simulink library "HEMERO"  (Simulink 3.00)
values from neighbouring files (symbols this model uses):
  K1 = 0.5    [ejh64.m]    (also in ejh65.m)
  K2 = 0.8    [ejh64.m]    (also in ejh65.m)
  x_camino = 0:0.01:10    [ejh64.m]    (also in ejh65.m)
  y_camino = x_camino.^2    [ejh64.m]    (also in ejh65.m)
undefined symbols (not defined in the file or in its folder): magnitude, nonlinear
libraries: simulink_extras x12, HEMERO x9, simulink3 x6, dspstat x4
(part 1 of 9)
settings Model: LastModifiedBy=Administrador

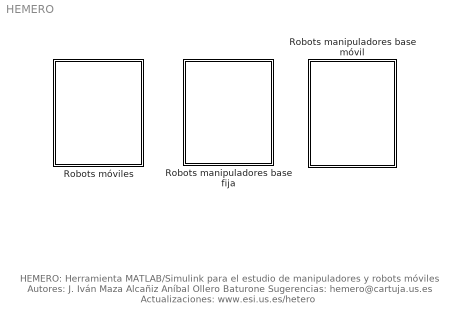
== system HEMERO ==
  note: HEMERO: Herramienta MATLAB/Simulink para el estudio de
      | manipuladores y robots móviles
      | Autores:
      | J. Iván Maza Alcañiz
      | Aníbal Ollero Baturone
      |
      | Sugerencias: hemero@cartuja.us.es
      | Actualizaciones: www.esi.us.es/hetero
  Robots manipuladores base fija : Subsystem
  Robots manipuladores base móvil : Subsystem
  Robots móviles : Subsystem

== system HEMERO/Robots manipuladores base fija ==
  Control basado en el modelo : Subsystem
  Modelo Dinámico : Subsystem

== system HEMERO/Robots manipuladores base móvil ==
  Modelo Dinámico : Subsystem

== system HEMERO/Robots móviles ==
  Control de robots móviles : Subsystem
  Modelos cinemáticos directos : Subsystem
  Modelos cinemáticos inversos : Subsystem

== system HEMERO/Robots manipuladores base fija/Control basado en el modelo ==
  Control Adaptativo : Subsystem
  Control con aprendizaje : Subsystem
  Par Computado : Subsystem

== system HEMERO/Robots manipuladores base fija/Modelo Dinámico ==
  Ejemplos : Subsystem
  Inversa de la matriz de masas : Subsystem  mask(Inversa de la matriz de masas){dyn=}
      mask prompts: dyn "Matriz de parámetros cinemáticos y dinámicos:"
      mask help: Este bloque calcula el producto de la inversa de la matriz de masas por el vector columna In que se le pasa como entrada.
  Modelo de fricciones : Subsystem  mask(Modelo de fricciones (viscosa y de Coriolis)){G=, b=, tcp=, tcm=}
      mask prompts: G "Factores de reducción (G):"; b "Fricciones viscosas, referidas al motor:"; tcp "Fricciones de Coulomb (rotación +), referidas al motor:"; tcm "Fricciones de Coulomb (rotación -), referidas al motor:"
      mask help:
      | Este bloque calcula el par correspondiente a la fricciones viscosa y de Coulomb. Para ello se emplea un determinado modelo para dichas fricciones:
      |            B·q' + Tc + ,  si q'>0
      |            B·q' + Tc - ,  si q'<0
      mask Display:
      | disp('B·q'' + Tc + ,  si q''>0\n')
      | disp('\nB·q'' + Tc - ,  si q''<0')
  Par total : Subsystem  mask(Par total){dyn=, grav=}
      mask prompts: dyn "Matriz de parámetros cinemáticos y dinámicos:"; grav "Vector aceleración de la gravedad:"
      mask help: Este bloque calcula el par total. Se incluye un modelo de las fricciones igual al empleado en el bloque "Modelo de fricciones". Si se quiere eliminar este término de fricciones para usar un modelo distinto, basta con hacer nulas las columnas 18, 19 y 20 de la matriz de parámetros cinemáticos y dinámicos.
  Trayectorias articulares : Subsystem  mask(Trayectorias articulares){dyn=, grav=, inivel=, inipos=}
      mask prompts: dyn "Matriz de parámetros cinemáticos y dinámicos:"; grav "Vector aceleración de la gravedad:"; inivel "Velocidades articulares iniciales:"; inipos "Posiciones articulares iniciales:"
      mask help: Se calculan las trayectorias articulares (posiciones, velocidades y aceleraciones articulares) a partir de los pares aplicados al manipulador.
  Término Vm de Coriolis : Subsystem  mask(Producto por el término Vm){dyn=}
      mask prompts: dyn "Matriz de parámetros cinemáticos y dinámicos:"
      mask help: Este bloque calcula el producto del término Vm por el vector columna In que se le pasa como entrada.
  Término de la matriz de masas : Subsystem  mask(Término asociado a la matriz de masas){dyn=}
      mask prompts: dyn "Matriz de parámetros cinemáticos y dinámicos:"
      mask help: Este bloque calcula el par correspondiente al término en el que aparece la matriz de masas.
  Términos gravitatorios : Subsystem  mask(Término gravitatorio){dyn=, grav=}
      mask prompts: dyn "Matriz de parámetros cinemáticos y dinámicos:"; grav "Vector aceleración de la gravedad:"
      mask help: Este bloque calcula el par correspondiente al término gravitatorio.
  Términos centrífugos y de Coriolis : Subsystem  mask(Términos centrífugos y de Coriolis){dyn=}
      mask prompts: dyn "Matriz de parámetros cinemáticos y dinámicos:"
      mask help: Este bloque calcula el par correspondiente a los términos centrífugos y de Coriolis.

== system HEMERO/Robots manipuladores base móvil/Modelo Dinámico ==
  Ejemplos : Subsystem
  Inversa de la matriz de masas : Subsystem  mask(Inversa de la matriz de masas){dyn=}
      mask prompts: dyn "Matriz de parámetros cinemáticos y dinámicos:"
      mask help: Este bloque calcula el producto de la inversa de la matriz de masas por el vector columna In que se le pasa como entrada, para el caso de base móvil.
  Modelo de fricciones : Subsystem  mask(Modelo de fricciones (viscosa y de Coriolis)){G=, b=, tcp=, tcm=}
      mask prompts: G "Factores de reducción (G):"; b "Fricciones viscosas, referidas al motor:"; tcp "Fricciones de Coulomb (rotación +), referidas al motor:"; tcm "Fricciones de Coulomb (rotación -), referidas al motor:"
      mask help:
      | Este bloque calcula el par correspondiente a la fricciones viscosa y de Coulomb. Para ello se emplea un determinado modelo para dichas fricciones:
      |            B·q' + Tc + ,  si q'>0
      |            B·q' + Tc - ,  si q'<0
      mask Display:
      | disp('B·q'' + Tc + ,  si q''>0\n')
      | disp('\nB·q'' + Tc - ,  si q''<0')
  Par total : Subsystem  mask(Par total){dyn=, grav=}
      mask prompts: dyn "Matriz de parámetros cinemáticos y dinámicos:"; grav "Vector aceleración de la gravedad:"
      mask help: Este bloque calcula el par total para el caso de base móvil. Se incluye un modelo de las fricciones igual al empleado en el bloque "Modelo de fricciones". Si se quiere eliminar este término de fricciones para usar un modelo distinto, basta con hacer nulas las columnas 18, 19 y 20 de la matriz de parámetros cinemáticos y dinámicos.
  Trayectorias articulares : Subsystem  mask(Trayectorias articulares){dyn=, grav=, inivel=, inipos=}
      mask prompts: dyn "Matriz de parámetros cinemáticos y dinámicos:"; grav "Vector aceleración de la gravedad:"; inivel "Velocidades articulares iniciales:"; inipos "Posiciones articulares iniciales:"
      mask help: Calcula las trayectorias articulares (posiciones, velocidades y aceleraciones articulares) a partir de los pares aplicados al manipulador, para el caso de base móvil.
  Término Vm de Coriolis : Subsystem  mask(Producto por el término Vm){dyn=}
      mask prompts: dyn "Matriz de parámetros cinemáticos y dinámicos:"
      mask help: Este bloque calcula el producto del término Vm por el vector columna In que se le pasa como entrada, para el caso de base móvil.
  Término de la matriz de masas : Subsystem  mask(Término asociado a la matriz de masas){dyn=}
      mask prompts: dyn "Matriz de parámetros cinemáticos y dinámicos:"
      mask help: Este bloque calcula el par correspondiente al término en el que aparece la matriz de masas para el caso de base móvil.
  Términos gravitatorios : Subsystem  mask(Término gravitatorio){dyn=, grav=}
      mask prompts: dyn "Matriz de parámetros cinemáticos y dinámicos:"; grav "Vector aceleración de la gravedad:"
      mask help: Este bloque calcula el par correspondiente al término gravitatorio para el caso de base móvil.
  Términos centrífugos y de Coriolis : Subsystem  mask(Términos centrífugos y de Coriolis){dyn=}
      mask prompts: dyn "Matriz de parámetros cinemáticos y dinámicos:"
      mask help: Este bloque calcula el par correspondiente a los términos centrífugos y de Coriolis para el caso de base móvil.

== system HEMERO/Robots móviles/Control de robots móviles ==
  Métodos geométricos : Subsystem
  Métodos basados en Teoría de Control : Subsystem

== system HEMERO/Robots móviles/Modelos cinemáticos directos ==
  Modelo directo Bicicleta : Subsystem  mask(Modelo directo bicicleta){x_ini=, y_ini=, phi_ini=, alpha_ini=, c=, l=}
      mask prompts: x_ini "Coordenada x inicial del móvil:"; y_ini "Coordenada y inicial del móvil:"; phi_ini "Valor inicial de la orientación del vehículo (rad):"; alpha_ini "Valor inicial de la orientación de la rueda delantera (rad):"; c "Radio de las ruedas"; l "Longitud entre rueda delantera y trasera:"
      mask help: Calcula las coordenadas y orientación del vehículo a partir de las variables de control wt (velocidad angular de rotación de la rueda delantera sobre si misma) y walpha (velocidad angular de giro de la rueda delantera).
  Modelo directo Config. Síncrona : Subsystem  mask(Modelo directo config. síncrona){x_ini=, y_ini=, phi_ini=}
      mask prompts: x_ini "Coordenada x inicial del móvil:"; y_ini "Coordenada y inicial del móvil:"; phi_ini "Valor inicial de la orientación del vehículo (rad):"
      mask help: Calcula las coordenadas y orientación del vehículo a partir de las variables de control v y w que son las velocidades lineal y angular respectivamente del vehículo.
  Modelo directo Guiado Diferencial : Subsystem  mask(Modelo directo guiado diferencial){x_ini=, y_ini=, phi_ini=, c=, b=}
      mask prompts: x_ini "Coordenada x inicial del móvil:"; y_ini "Coordenada y inicial del móvil:"; phi_ini "Valor inicial de la orientación del vehículo (rad):"; c "Radio de las ruedas:"; b "Distancia entre las ruedas :"
      mask help: Calcula las coordenadas y orientación del vehículo a partir de las variables de control wi y wd que son las velocidades angulares de las ruedas izquierda y derecha respectivamente.
  Modelo directo Triciclo Clásico : Subsystem  mask(Modelo directo triciclo clásico){x_ini=, y_ini=, phi_ini=, alpha_ini=, c=, l=}
      mask prompts: x_ini "Coordenada x inicial del móvil:"; y_ini "Coordenada y inicial del móvil:"; phi_ini "Valor inicial de la orientación del vehículo (rad):"; alpha_ini "Valor inicial de la orientación de la rueda delantera (rad):"; c "Radio de las ruedas"; l "Longitud entre rueda delantera y traseras:"
      mask help: Calcula las coordenadas y orientación del vehículo a partir de las variables de control wt (velocidad angular de rotación de la rueda delantera sobre si misma) y walpha (velocidad angular de giro de la rueda delantera).

== system HEMERO/Robots móviles/Modelos cinemáticos inversos ==
  Modelo inverso Bicicleta : Subsystem  mask(Modelo inverso de la bicicleta){l=}
      mask prompts: l "Distancia entre la rueda delantera y la rueda trasera:"
      mask help: A partir de las coordenadas (x,y) de la trayectoria de la bicicleta en función del tiempo, este bloque calcula las correspondientes variables de control vt (velocidad lineal de la rueda delantera) y walpha (velocidad angular de giro de la rueda delantera). Asimismo, también calcula el ángulo (alpha) de orientación de la rueda delantera y el ángulo (phi) de orientación del vehículo.
  Modelo inverso Config. Síncrona : Subsystem
      mask Type: Modelo inverso de la configuración síncrona
      mask Description: A partir de las coordenadas (x,y) de la trayectoria del vehículo en función del tiempo, este bloque calcula las correspondientes variables de control v y w que son las velocidades lineal y angular del vehículo. Asimismo, también se calcula la orientación (phi) del vehículo.
  Modelo inverso Guiado Diferencial : Subsystem  mask(Modelo inverso guiado diferencial){b=, c=}
      mask prompts: b "Vía del vehículo:"; c "Radio de las ruedas:"
      mask help: A partir de las coordenadas (x,y) de la trayectoria del vehículo en función del tiempo, este bloque calcula las correspondientes variables de control wi y wd que son las velocidades angulares de giro de las ruedas izquierda y derecha respectivamente.
  Modelo inverso Triciclo Clasico : Subsystem  mask(Modelo inverso del triciclo clasico){l=}
      mask prompts: l "Distancia entre la rueda delantera y las ruedas traseras:"
      mask help: A partir de las coordenadas (x,y) de la trayectoria del triciclo en función del tiempo, este bloque calcula las correspondientes variables de control vt (velocidad lineal de la rueda delantera) y walpha (velocidad angular de giro de la rueda delantera). Asimismo, también calcula el ángulo (alpha) de orientación de la rueda delantera y el ángulo (phi) de orientación del vehículo.

== system HEMERO/Robots manipuladores base fija/Control basado en el modelo/Control Adaptativo ==
  Control de inercia adaptativo : Subsystem  mask(Cálcula los parámetros para el control de inercia adaptativo){dyn=, gamma=, a=, grav=, m_inicial=, b_inicial=, tcp_inicial=, tcm_inicial=}
      mask prompts: dyn "Matriz de parámetros cinemáticos y dinámicos:"; gamma "Matriz gamma:"; a "Matriz A:"; grav "Vector aceleración de la gravedad:"; m_inicial "Estimaciones de las masas:"; b_inicial "Estimaciones de las fricciones viscosas:"; tcp_inicial "Estimaciones de las fricciones de Coulomb (rotación +):"; tcm_inicial "Estimaciones de las fricciones de Coulomb (rotación -):"
      mask help: Este bloque calcula en cada instante las estimaciones de las masas y fricciones de un manipulador según el esquema de control de inercia adaptativo. Asimismo, devuelve el término Y(·)*estim correspondiente a uno de los sumandos que componen el par de control en dicho esquema.
  Ejemplos : Subsystem
  Inversa de la matriz de masas : Subsystem  mask(Inversa de la matriz de masas){dyn=}
      mask prompts: dyn "Matriz de parámetros cinemáticos y dinámicos:"
      mask help: Este bloque calcula el producto de la inversa de la matriz de masas por el vector columna In que se le pasa como entrada. Dispone de una entrada para proporcionarle las estimaciones de las masas en cada instante.
      mask Display:
      | plot([0.05 0.95],[0.05 0.95])
      | plot([0.8 0.95],[0.7 0.95])
      | plot([0.7 0.95],[0.8 0.95])
  Modelo de fricciones : Subsystem  mask(Modelo estimado de fricciones (viscosa y de Coriolis)){G=, b=, tcp=, tcm=}
      mask prompts: G "Factores de reducción (G):"; b "Fricciones viscosas iniciales, referidas al motor:"; tcp "Fricciones de Coulomb (rot +) iniciales, referidas al motor:"; tcm "Fricciones de Coulomb (rot -) iniciales, referidas al motor:"
      mask help:
      | Este bloque calcula el par correspondiente a la fricciones viscosa y de Coulomb. Para ello se emplea un determinado modelo para dichas fricciones:
      |            b·q' + tcp ,  si q'>0
      |            b·q' + tcm ,  si q'<0
      | Dispone de entradas para pasarle las estimaciones de las fricciones en cada instante.
      mask Display:
      | disp('B·q'' + Tc + ,  si q''>0\n')
      | disp('\nB·q'' + Tc - ,  si q''<0')
      | plot([0.05 0.95],[0.05 0.95])
      | plot([0.8 0.95],[0.7 0.95])
      | plot([0.78 0.95],[0.88 0.95])
  Término Vm de Coriolis : Subsystem  mask(Término estimado asociado a la matriz de masas){dyn=}
      mask prompts: dyn "Matriz inicial de parámetros cinemáticos y dinámicos:"
      mask help: Este bloque calcula el par correspondiente al término en el que aparece la matriz de masas. Dispone de una entrada para proporcionarle las estimaciones de las masas en cada instante.
      mask Display:
      | plot([0.05 0.95],[0.05 0.95])
      | plot([0.8 0.95],[0.7 0.95])
      | plot([0.7 0.95],[0.8 0.95])
  Término de la matriz de masas : Subsystem  mask(Término estimado asociado a la matriz de masas){dyn=}
      mask prompts: dyn "Matriz inicial de parámetros cinemáticos y dinámicos:"
      mask help: Este bloque calcula el par correspondiente al término en el que aparece la matriz de masas. Dispone de una entrada para proporcionarle las estimaciones de las masas en cada instante.
      mask Display:
      | plot([0.05 0.95],[0.05 0.95])
      | plot([0.8 0.95],[0.7 0.95])
      | plot([0.7 0.95],[0.8 0.95])
  Términos gravitatorios : Subsystem  mask(Término gravitatorio estimado){dyn=, grav=}
      mask prompts: dyn "Matriz inicial de parámetros cinemáticos y dinámicos:"; grav "Vector aceleración de la gravedad:"
      mask help: Este bloque calcula el par correspondiente al término gravitatorio. Dispone de una entrada para proporcionarle las estimaciones de las masas en cada instante.
      mask Display:
      | plot([0.05 0.95],[0.05 0.95])
      | plot([0.8 0.95],[0.7 0.95])
      | plot([0.7 0.95],[0.8 0.95])
  Términos centrífugos y de Coriolis : Subsystem  mask(Términos centrífugos y de Coriolis estimados){dyn=}
      mask prompts: dyn "Matriz inicial de parámetros cinemáticos y dinámicos:"
      mask help: Este bloque calcula el par correspondiente a los términos centrífugos y de Coriolis. Dispone de una entrada para proporcionarle las estimaciones de las masas en cada instante.
      mask Display:
      | plot([0.05 0.95],[0.05 0.95])
      | plot([0.8 0.95],[0.7 0.95])
      | plot([0.7 0.95],[0.8 0.95])

== system HEMERO/Robots manipuladores base fija/Control basado en el modelo/Control con aprendizaje ==
  Ejemplos : Subsystem
  Par realimentado aprendido : Subsystem  mask(Calcula por aprendizaje el par que hay que añadir a la ley de control){dyn=, Kp=, Kv=, mu=, tfinal=}
      mask prompts: dyn "Matriz de parámetros cinemáticos y dinámicos:"; Kp "Matriz Kp:"; Kv "Matriz Kv:"; mu "Constante mu:"; tfinal "Tiempo final de la simulación:"

== system HEMERO/Robots manipuladores base fija/Control basado en el modelo/Par Computado ==
  Control PD : Subsystem  mask(Controlador PD){Kp=, Kv=}
      mask prompts: Kp "Introduzca la matriz Kp:"; Kv "Introduzca la matriz Kv:"
      mask help: Calcula el par tau_r correspondiente a la técnica del par computado usando un controlador PD.
  Control PID : Subsystem  mask(Controlador PID){Kp=, Kv=, Ki=}
      mask prompts: Kp "Introduzca la matriz Kp:"; Kv "Introduzca la matriz Kv:"; Ki "Introduzca la matriz Ki:"
      mask help: Calcula el par tau_r correspondiente a la técnica del par computado usando un controlador PID.
  Ejemplos : Subsystem

== system HEMERO/Robots manipuladores base fija/Modelo Dinámico/Ejemplos ==
  Ejemplo H.4.2 : Subsystem
  Ejemplo H.4.4a : Subsystem
  Ejemplo H.4.4b : Subsystem
  Ejemplo H.4.4c : Subsystem

== system HEMERO/Robots manipuladores base fija/Modelo Dinámico/Inversa de la matriz de masas ==
  q : Inport  Port=1  PortWidth=-1  SampleTime=-1  DataType=auto
      settings: SignalType=auto
  In : Inport  Port=2  PortWidth=-1  SampleTime=-1  DataType=auto
      settings: SignalType=auto
  Masas : S-Function  FunctionName=sminv  Parameters=dyn  PortCounts=[]  SFunctionModules=''
  Mux : Mux  Inputs=2
      settings: DisplayOption=none
  M(q)^(-1) · In : Outport  Port=1  InitialOutput=0
  wires:
  Masas/1 -> M(q)^(-1) · In/1
  In/1 -> Mux/2
  q/1 -> Mux/1
  Mux/1 -> Masas/1

== system HEMERO/Robots manipuladores base fija/Modelo Dinámico/Modelo de fricciones ==
  q' : Inport  Port=1  PortWidth=-1  SampleTime=-1  DataType=auto
      settings: SignalType=auto
  Fricciones : S-Function  FunctionName=sfriction  Parameters=G,b,tcp,tcm  PortCounts=[]  SFunctionModules=''
  tau_f : Outport  Port=1  InitialOutput=0
  wires:
  Fricciones/1 -> tau_f/1
  q'/1 -> Fricciones/1

== system HEMERO/Robots manipuladores base fija/Modelo Dinámico/Par total ==
  q : Inport  Port=1  PortWidth=-1  SampleTime=-1  DataType=auto
      settings: SignalType=auto
  q' : Inport  Port=2  PortWidth=-1  SampleTime=-1  DataType=auto
      settings: SignalType=auto
  q'' : Inport  Port=3  PortWidth=-1  SampleTime=-1  DataType=auto
      settings: SignalType=auto
  fext : Inport  Port=4  PortWidth=-1  SampleTime=-1  DataType=auto
      settings: SignalType=auto
  Mux : Mux  Inputs=4
      settings: DisplayOption=none
  Par total : S-Function  FunctionName=srne  Parameters=dyn,grav  PortCounts=[]  SFunctionModules=''
  M(q)·q'' + V (q,q') + G(q) + F(q') : Outport  Port=1  InitialOutput=0
  wires:
  Par total/1 -> M(q)·q'' + V (q,q') + G(q) + F(q')/1
  Mux/1 -> Par total/1
  q''/1 -> Mux/3
  q'/1 -> Mux/2
  q/1 -> Mux/1
  fext/1 -> Mux/4

== system HEMERO/Robots manipuladores base fija/Modelo Dinámico/Trayectorias articulares ==
  note: q
  note: q''
  note: q'
  tau : Inport  Port=1  PortWidth=-1  SampleTime=-1  DataType=auto
      settings: SignalType=auto
  Integrator : Integrator  ExternalReset=none  InitialConditionSource=internal  InitialCondition=inivel(:)  LimitOutput=off  UpperSaturationLimit=inf  LowerSaturationLimit=-inf  ShowSaturationPort=off  ShowStatePort=off  AbsoluteTolerance=auto
  Integrator1 : Integrator  ExternalReset=none  InitialConditionSource=internal  InitialCondition=inipos(:)  LimitOutput=off  UpperSaturationLimit=inf  LowerSaturationLimit=-inf  ShowSaturationPort=off  ShowStatePort=off  AbsoluteTolerance=auto
  Inversa de la matriz de masas : Subsystem  mask(Término de Coriolis){dyn=dyn}
      mask prompts: dyn "Matriz de parámetros dinámicos:"
      mask help: Este bloque devuelve el par correspondiente al término de Coriolis.
      mask Help: A este bloque hay que darle tres parámetros: 1) La matriz de parámetros dinámicos del manipulador de acuerdo con el formato que se explica en la sección "dyn" del Apéndice, 2) Un vector columna correspondiente a la aceleración de la gravedad, y 3) Un vector columna correspondiente a las fuerzas externas.
  Modelo de fricciones : Subsystem  mask(Modelo de fricciones (viscosa y de Coriolis)){G=dyn (:,17), b=dyn (:,18), tcp=dyn (:,19), tcm=dyn (:,20)}
      mask prompts: G "Factores de reducción (G):"; b "Fricciones viscosas, referidas al motor:"; tcp "Fricciones de Coulomb (rotación +), referidas al motor:"; tcm "Fricciones de Coulomb (rotación -), referidas al motor:"
      mask help:
      | Este bloque calcula el par correspondiente a la fricciones viscosa y de Coulomb. Para ello se emplea un determinado modelo para dichas fricciones:
      |            B·q' + Tc + ,  si q'>0
      |            B·q' + Tc - ,  si q'<0
      mask Display:
      | disp('B·q'' + Tc + ,  si q''>0\n')
      | disp('\nB·q'' + Tc - ,  si q''<0')
  Sum : Sum  Inputs=+---  SaturateOnIntegerOverflow=on
  Términos gravitatorios : Subsystem  mask(Término de Coriolis){dyn=dyn, grav=grav}
      mask prompts: dyn "Matriz de parámetros dinámicos:"; grav "Vector aceleración de la gravedad:"
      mask help: Este bloque devuelve el par correspondiente al término de Coriolis.
      mask Help: A este bloque hay que darle tres parámetros: 1) La matriz de parámetros dinámicos del manipulador de acuerdo con el formato que se explica en la sección "dyn" del Apéndice, 2) Un vector columna correspondiente a la aceleración de la gravedad, y 3) Un vector columna correspondiente a las fuerzas externas.
  Términos centrífugos y de Coriolis : Subsystem  mask(Término de Coriolis){dyn=dyn}
      mask prompts: dyn "Matriz de parámetros dinámicos:"
      mask help: Este bloque devuelve el par correspondiente al término de Coriolis.
      mask Help: A este bloque hay que darle tres parámetros: 1) La matriz de parámetros dinámicos del manipulador de acuerdo con el formato que se explica en la sección "dyn" del Apéndice, 2) Un vector columna correspondiente a la aceleración de la gravedad, y 3) Un vector columna correspondiente a las fuerzas externas.
  q : Outport  Port=1  InitialOutput=0
  q' : Outport  Port=2  InitialOutput=0
  q'' : Outport  Port=3  InitialOutput=0
  wires:
  Integrator1/1 -> q/1, Inversa de la matriz de masas/1(q), Términos centrífugos y de Coriolis/1(q), Términos gravitatorios/1(q)
  Integrator/1 -> Integrator1/1, q'/1, Términos centrífugos y de Coriolis/2(q'), Modelo de fricciones/1(q')
  Sum/1 -> Inversa de la matriz de masas/2(In)
  tau/1 -> Sum/1
  Inversa de la matriz de masas/1(M(q)^(-1) · In) -> Integrator/1, q''/1
  Términos gravitatorios/1(G (q)) -> Sum/4
  Términos centrífugos y de Coriolis/1(V (q,q')) -> Sum/3
  Modelo de fricciones/1(tau_f) -> Sum/2

== system HEMERO/Robots manipuladores base fija/Modelo Dinámico/Término Vm de Coriolis ==
  q : Inport  Port=1  PortWidth=-1  SampleTime=-1  DataType=auto
      settings: SignalType=auto
  q' : Inport  Port=2  PortWidth=-1  SampleTime=-1  DataType=auto
      settings: SignalType=auto
  In : Inport  Port=3  PortWidth=-1  SampleTime=-1  DataType=auto
      settings: SignalType=auto
  " " : S-Function  FunctionName=svmcorioli  Parameters=dyn  PortCounts=[]  SFunctionModules=''
  Mux : Mux  Inputs=3
      settings: DisplayOption=none
  Vm(q,q') · In : Outport  Port=1  InitialOutput=0
  wires:
  q'/1 -> Mux/2
  q/1 -> Mux/1
  In/1 -> Mux/3
  " "/1 -> Vm(q,q') · In/1
  Mux/1 -> " "/1

== system HEMERO/Robots manipuladores base fija/Modelo Dinámico/Término de la matriz de masas ==
  q : Inport  Port=1  PortWidth=-1  SampleTime=-1  DataType=auto
      settings: SignalType=auto
  In : Inport  Port=2  PortWidth=-1  SampleTime=-1  DataType=auto
      settings: SignalType=auto
  Masas : S-Function  FunctionName=sinertia  Parameters=dyn  PortCounts=[]  SFunctionModules=''
  Mux : Mux  Inputs=2
      settings: DisplayOption=none
  M (q)·In : Outport  Port=1  InitialOutput=0
  wires:
  Masas/1 -> M (q)·In/1
  In/1 -> Mux/2
  q/1 -> Mux/1
  Mux/1 -> Masas/1

== system HEMERO/Robots manipuladores base fija/Modelo Dinámico/Términos gravitatorios ==
  q : Inport  Port=1  PortWidth=-1  SampleTime=-1  DataType=auto
      settings: SignalType=auto
  Gravedad : S-Function  FunctionName=sgravity  Parameters=dyn,grav  PortCounts=[]  SFunctionModules=''
  G (q) : Outport  Port=1  InitialOutput=0
  wires:
  Gravedad/1 -> G (q)/1
  q/1 -> Gravedad/1

== system HEMERO/Robots manipuladores base fija/Modelo Dinámico/Términos centrífugos y de Coriolis ==
  q : Inport  Port=1  PortWidth=-1  SampleTime=-1  DataType=auto
      settings: SignalType=auto
  q' : Inport  Port=2  PortWidth=-1  SampleTime=-1  DataType=auto
      settings: SignalType=auto
  Centrífugos y Coriolis : S-Function  FunctionName=scoriolis  Parameters=dyn  PortCounts=[]  SFunctionModules=''
  Mux : Mux  Inputs=2
      settings: DisplayOption=none
  V (q,q') : Outport  Port=1  InitialOutput=0
  wires:
  Centrífugos y Coriolis/1 -> V (q,q')/1
  q'/1 -> Mux/2
  q/1 -> Mux/1
  Mux/1 -> Centrífugos y Coriolis/1

== system HEMERO/Robots manipuladores base móvil/Modelo Dinámico/Ejemplos ==

== system HEMERO/Robots manipuladores base móvil/Modelo Dinámico/Inversa de la matriz de masas ==
  q : Inport  Port=1  PortWidth=-1  SampleTime=-1  DataType=auto
      settings: SignalType=auto
  In : Inport  Port=2  PortWidth=-1  SampleTime=-1  DataType=auto
      settings: SignalType=auto
  w0 : Inport  Port=3  PortWidth=-1  SampleTime=-1  DataType=auto
      settings: SignalType=auto
  w0 ' : Inport  Port=4  PortWidth=-1  SampleTime=-1  DataType=auto
      settings: SignalType=auto
  v0 ' : Inport  Port=5  PortWidth=-1  SampleTime=-1  DataType=auto
      settings: SignalType=auto
  Masas : S-Function  FunctionName=msminv  Parameters=dyn  PortCounts=[]  SFunctionModules=''
  Mux : Mux  Inputs=5
      settings: DisplayOption=none
  M(q)^(-1) · In : Outport  Port=1  InitialOutput=0
  wires:
  Mux/1 -> Masas/1
  q/1 -> Mux/1
  In/1 -> Mux/2
  Masas/1 -> M(q)^(-1) · In/1
  w0/1 -> Mux/3
  v0 '/1 -> Mux/5
  w0 '/1 -> Mux/4

== system HEMERO/Robots manipuladores base móvil/Modelo Dinámico/Modelo de fricciones ==
  q' : Inport  Port=1  PortWidth=-1  SampleTime=-1  DataType=auto
      settings: SignalType=auto
  Fricciones : S-Function  FunctionName=sfriction  Parameters=G,b,tcp,tcm  PortCounts=[]  SFunctionModules=''
  tau_f : Outport  Port=1  InitialOutput=0
  wires:
  q'/1 -> Fricciones/1
  Fricciones/1 -> tau_f/1

== system HEMERO/Robots manipuladores base móvil/Modelo Dinámico/Par total ==
  q : Inport  Port=1  PortWidth=-1  SampleTime=-1  DataType=auto
      settings: SignalType=auto
  q' : Inport  Port=2  PortWidth=-1  SampleTime=-1  DataType=auto
      settings: SignalType=auto
  q'' : Inport  Port=3  PortWidth=-1  SampleTime=-1  DataType=auto
      settings: SignalType=auto
  fext : Inport  Port=4  PortWidth=-1  SampleTime=-1  DataType=auto
      settings: SignalType=auto
  w0 : Inport  Port=5  PortWidth=-1  SampleTime=-1  DataType=auto
      settings: SignalType=auto
  w0 ' : Inport  Port=6  PortWidth=-1  SampleTime=-1  DataType=auto
      settings: SignalType=auto
  v0 ' : Inport  Port=7  PortWidth=-1  SampleTime=-1  DataType=auto
      settings: SignalType=auto
  Mux : Mux  Inputs=7
      settings: DisplayOption=none
  Par total : S-Function  FunctionName=msrne  Parameters=dyn,grav  PortCounts=[]  SFunctionModules=''
  M(q)·q'' + V (q,q') + G(q) + F(q') : Outport  Port=1  InitialOutput=0
  wires:
  fext/1 -> Mux/4
  q/1 -> Mux/1
  q'/1 -> Mux/2
  q''/1 -> Mux/3
  Mux/1 -> Par total/1
  Par total/1 -> M(q)·q'' + V (q,q') + G(q) + F(q')/1
  w0/1 -> Mux/5
  w0 '/1 -> Mux/6
  v0 '/1 -> Mux/7

== system HEMERO/Robots manipuladores base móvil/Modelo Dinámico/Trayectorias articulares ==
  tau : Inport  Port=1  PortWidth=-1  SampleTime=-1  DataType=auto
      settings: SignalType=auto
  w0 : Inport  Port=2  PortWidth=-1  SampleTime=-1  DataType=auto
      settings: SignalType=auto
  w0 ' : Inport  Port=3  PortWidth=-1  SampleTime=-1  DataType=auto
      settings: SignalType=auto
  v0 ' : Inport  Port=4  PortWidth=-1  SampleTime=-1  DataType=auto
      settings: SignalType=auto
  Integrator : Integrator  ExternalReset=none  InitialConditionSource=internal  InitialCondition=inivel(:)  LimitOutput=off  UpperSaturationLimit=inf  LowerSaturationLimit=-inf  ShowSaturationPort=off  ShowStatePort=off  AbsoluteTolerance=auto
  Integrator1 : Integrator  ExternalReset=none  InitialConditionSource=internal  InitialCondition=inipos(:)  LimitOutput=off  UpperSaturationLimit=inf  LowerSaturationLimit=-inf  ShowSaturationPort=off  ShowStatePort=off  AbsoluteTolerance=auto
  Inversa de la matriz de masas : Subsystem  mask(Inversa de la matriz de masas){dyn=dyn}
      mask prompts: dyn "Matriz de parámetros cinemáticos y dinámicos:"
      mask help: Este bloque calcula el producto de la inversa de la matriz de masas por el vector columna In que se le pasa como entrada.
  Modelo de fricciones : Subsystem  mask(Modelo de fricciones (viscosa y de Coriolis)){G=dyn (:,17), b=dyn (:,18), tcp=dyn (:,19), tcm=dyn (:,20)}
      mask prompts: G "Factores de reducción (G):"; b "Fricciones viscosas, referidas al motor:"; tcp "Fricciones de Coulomb (rotación +), referidas al motor:"; tcm "Fricciones de Coulomb (rotación -), referidas al motor:"
      mask help:
      | Este bloque calcula el par correspondiente a la fricciones viscosa y de Coulomb. Para ello se emplea un determinado modelo para dichas fricciones:
      |            B·q' + Tc + ,  si q'>0
      |            B·q' + Tc - ,  si q'<0
      mask Display:
      | disp('B·q'' + Tc + ,  si q''>0\n')
      | disp('\nB·q'' + Tc - ,  si q''<0')
  Sum : Sum  Inputs=+---  SaturateOnIntegerOverflow=on
  Términos gravitatorios : Subsystem  mask(Término gravitatorio){dyn=dyn, grav=grav}
      mask prompts: dyn "Matriz de parámetros cinemáticos y dinámicos:"; grav "Vector aceleración de la gravedad:"
      mask help: Este bloque calcula el par correspondiente al término gravitatorio para el caso de base móvil.
  Términos centrífugos y de Coriolis : Subsystem  mask(Términos centrífugos y de Coriolis){dyn=dyn}
      mask prompts: dyn "Matriz de parámetros cinemáticos y dinámicos:"
      mask help: Este bloque calcula el par correspondiente a los términos centrífugos y de Coriolis para el caso de base móvil.
  q : Outport  Port=1  InitialOutput=0
  q' : Outport  Port=2  InitialOutput=0
  q'' : Outport  Port=3  InitialOutput=0
  wires:
  Modelo de fricciones/1(tau_f) -> Sum/2
  tau/1 -> Sum/1
  Integrator/1 -> Modelo de fricciones/1(q'), Términos centrífugos y de Coriolis/2(q'), q'/1, Integrator1/1
  Integrator1/1 -> Términos gravitatorios/1(q), Términos centrífugos y de Coriolis/1(q), Inversa de la matriz de masas/1(q), q/1
  Términos centrífugos y de Coriolis/1(V (q,q')) -> Sum/3
  Términos gravitatorios/1(G (q)) -> Sum/4
  Sum/1 -> Inversa de la matriz de masas/2(In)
  Inversa de la matriz de masas/1(M(q)^(-1) · In) -> q''/1, Integrator/1
  v0 '/1 -> Términos gravitatorios/4(v0 '), Términos centrífugos y de Coriolis/5(v0 '), Inversa de la matriz de masas/5(v0 ')
  w0 '/1 -> Términos centrífugos y de Coriolis/4(w0 '), Términos gravitatorios/3(w0 '), Inversa de la matriz de masas/4(w0 ')
  w0/1 -> Términos centrífugos y de Coriolis/3(w0), Términos gravitatorios/2(w0), Inversa de la matriz de masas/3(w0)

== system HEMERO/Robots manipuladores base móvil/Modelo Dinámico/Término Vm de Coriolis ==
  q : Inport  Port=1  PortWidth=-1  SampleTime=-1  DataType=auto
      settings: SignalType=auto
  q' : Inport  Port=2  PortWidth=-1  SampleTime=-1  DataType=auto
      settings: SignalType=auto
  In : Inport  Port=3  PortWidth=-1  SampleTime=-1  DataType=auto
      settings: SignalType=auto
  w0 : Inport  Port=4  PortWidth=-1  SampleTime=-1  DataType=auto
      settings: SignalType=auto
  w0 ' : Inport  Port=5  PortWidth=-1  SampleTime=-1  DataType=auto
      settings: SignalType=auto
  v0 ' : Inport  Port=6  PortWidth=-1  SampleTime=-1  DataType=auto
      settings: SignalType=auto
  " " : S-Function  FunctionName=mmcoriolis  Parameters=dyn  PortCounts=[]  SFunctionModules=''
  Mux : Mux  Inputs=6
      settings: DisplayOption=none
  Vm(q,q') · In : Outport  Port=1  InitialOutput=0
  wires:
  Mux/1 -> " "/1
  " "/1 -> Vm(q,q') · In/1
  In/1 -> Mux/3
  q/1 -> Mux/1
  q'/1 -> Mux/2
  w0/1 -> Mux/4
  w0 '/1 -> Mux/5
  v0 '/1 -> Mux/6

== system HEMERO/Robots manipuladores base móvil/Modelo Dinámico/Término de la matriz de masas ==
  q : Inport  Port=1  PortWidth=-1  SampleTime=-1  DataType=auto
      settings: SignalType=auto
  In : Inport  Port=2  PortWidth=-1  SampleTime=-1  DataType=auto
      settings: SignalType=auto
  w0 : Inport  Port=3  PortWidth=-1  SampleTime=-1  DataType=auto
      settings: SignalType=auto
  w0 ' : Inport  Port=4  PortWidth=-1  SampleTime=-1  DataType=auto
      settings: SignalType=auto
  v0 ' : Inport  Port=5  PortWidth=-1  SampleTime=-1  DataType=auto
      settings: SignalType=auto
  Masas : S-Function  FunctionName=msinertia  Parameters=dyn  PortCounts=[]  SFunctionModules=''
  Mux : Mux  Inputs=5
      settings: DisplayOption=none
  M (q)·In : Outport  Port=1  InitialOutput=0
  wires:
  Mux/1 -> Masas/1
  q/1 -> Mux/1
  In/1 -> Mux/2
  Masas/1 -> M (q)·In/1
  w0/1 -> Mux/3
  w0 '/1 -> Mux/4
  v0 '/1 -> Mux/5

== system HEMERO/Robots manipuladores base móvil/Modelo Dinámico/Términos gravitatorios ==
  q : Inport  Port=1  PortWidth=-1  SampleTime=-1  DataType=auto
      settings: SignalType=auto
  w0 : Inport  Port=2  PortWidth=-1  SampleTime=-1  DataType=auto
      settings: SignalType=auto
  w0 ' : Inport  Port=3  PortWidth=-1  SampleTime=-1  DataType=auto
      settings: SignalType=auto
  v0 ' : Inport  Port=4  PortWidth=-1  SampleTime=-1  DataType=auto
      settings: SignalType=auto
  Gravedad : S-Function  FunctionName=msgravity  Parameters=dyn,grav  PortCounts=[]  SFunctionModules=''
  Mux : Mux  Inputs=4
      settings: DisplayOption=none
  G (q) : Outport  Port=1  InitialOutput=0
  wires:
  q/1 -> Mux/1
  w0/1 -> Mux/2
  w0 '/1 -> Mux/3
  v0 '/1 -> Mux/4
  Mux/1 -> Gravedad/1
  Gravedad/1 -> G (q)/1

== system HEMERO/Robots manipuladores base móvil/Modelo Dinámico/Términos centrífugos y de Coriolis ==
  q : Inport  Port=1  PortWidth=-1  SampleTime=-1  DataType=auto
      settings: SignalType=auto
  q' : Inport  Port=2  PortWidth=-1  SampleTime=-1  DataType=auto
      settings: SignalType=auto
  w0 : Inport  Port=3  PortWidth=-1  SampleTime=-1  DataType=auto
      settings: SignalType=auto
  w0 ' : Inport  Port=4  PortWidth=-1  SampleTime=-1  DataType=auto
      settings: SignalType=auto
  v0 ' : Inport  Port=5  PortWidth=-1  SampleTime=-1  DataType=auto
      settings: SignalType=auto
  Centrífugos y Coriolis : S-Function  FunctionName=mscoriolis  Parameters=dyn  PortCounts=[]  SFunctionModules=''
  Mux : Mux  Inputs=5
      settings: DisplayOption=none
  V (q,q') : Outport  Port=1  InitialOutput=0
  wires:
  Mux/1 -> Centrífugos y Coriolis/1
  q/1 -> Mux/1
  q'/1 -> Mux/2
  Centrífugos y Coriolis/1 -> V (q,q')/1
  w0/1 -> Mux/3
  w0 '/1 -> Mux/4
  v0 '/1 -> Mux/5

== system HEMERO/Robots móviles/Control de robots móviles/Métodos geométricos ==
  Pure Pursuit I : Subsystem  mask(Pure Pursuit I){x_camino=, y_camino=, L=}
      mask prompts: x_camino "Coordenadas x del camino:"; y_camino "Coordenadas y del camino:"; L "Parámetro Look-ahead (L):"
      mask help: Este bloque se encarga de calcular la curvatura que es necesario suministrar al vehículo cuando se emplea la técnica de persecución pura con el parámetro look-ahead (L) fijo.
      mask init:
      | global K_ANT
      | K_ANT=1;
  Pure Pursuit II : Subsystem  mask(Pure Pursuit II){x_camino=, y_camino=, s=}
      mask prompts: x_camino "Coordenadas x del camino:"; y_camino "Coordenadas y del camino:"; s "Distancia sobre el camino (s):"
      mask help: Este bloque se encarga de calcular la curvatura que es necesario suministrar al vehículo cuando se emplea la técnica de persecución pura con el parámetro look-ahead (L) variable en función del punto objetivo.
      mask init:
      | global K_ANT
      | global INDEX
      | K_ANT=1;
      | for k=1:length(x_camino)-1
      |    acum(k)=0;
      |    for w=k:length(x_camino)-1
      |       dist_entre_puntos=sqrt( (x_camino(w)-x_camino(w+1))^2 + (y_camino(w)-y_camino(w+1))^2 );
      |       acum(w+1)=acum(w)+dist_entre_puntos;
      |    end
      |    dif=abs(acum-s);
      |    [z,indice] = min(dif);
      |    INDEX(k)=indice;
      | end
  Pure Pursuit III : Subsystem  mask(Pure Pursuit III){x_camino=, y_camino=, s=, Lmax=}
      mask prompts: x_camino "Coordenadas x del camino:"; y_camino "Coordenadas y del camino:"; s "Distancia sobre el camino (s):"; Lmax "Valor máximo de L:"
      mask help: Este bloque se encarga de calcular la curvatura que es necesario suministrar al vehículo cuando se emplea la técnica de persecución pura con el parámetro look-ahead (L) variable en función del punto objetivo. Es posible fijar un valor máximo para L.
      mask init: same as HEMERO/Robots móviles/Control de robots móviles/Métodos geométricos/Pure Pursuit II

== system HEMERO/Robots móviles/Control de robots móviles/Métodos basados en Teoría de Control ==
  Seguimiento de caminos : Subsystem
  Seguimiento de trayectorias : Subsystem

== system HEMERO/Robots móviles/Modelos cinemáticos directos/Modelo directo Bicicleta ==
  note: phi
  note: alpha
  note: vt
  wt : Inport  Port=1  PortWidth=-1  SampleTime=-1  DataType=auto
      settings: SignalType=auto
  walpha : Inport  Port=2  PortWidth=-1  SampleTime=-1  DataType=auto
      settings: SignalType=auto
  Gain : Gain  Gain=c  SaturateOnIntegerOverflow=on
  Gain1 : Gain  Orientation=up  Gain=1/l  SaturateOnIntegerOverflow=on
  Gain2 : Gain  Gain=-1  SaturateOnIntegerOverflow=on
  Integrator : Integrator  ExternalReset=none  InitialConditionSource=internal  InitialCondition=alpha_ini  LimitOutput=off  UpperSaturationLimit=inf  LowerSaturationLimit=-inf  ShowSaturationPort=off  ShowStatePort=off  AbsoluteTolerance=auto
  Integrator1 : Integrator  ExternalReset=none  InitialConditionSource=internal  InitialCondition=phi_ini  LimitOutput=off  UpperSaturationLimit=inf  LowerSaturationLimit=-inf  ShowSaturationPort=off  ShowStatePort=off  AbsoluteTolerance=auto
  Integrator2 : Integrator  ExternalReset=none  InitialConditionSource=internal  InitialCondition=x_ini  LimitOutput=off  UpperSaturationLimit=inf  LowerSaturationLimit=-inf  ShowSaturationPort=off  ShowStatePort=off  AbsoluteTolerance=auto
  Integrator3 : Integrator  ExternalReset=none  InitialConditionSource=internal  InitialCondition=y_ini  LimitOutput=off  UpperSaturationLimit=inf  LowerSaturationLimit=-inf  ShowSaturationPort=off  ShowStatePort=off  AbsoluteTolerance=auto
  Product{3..6} (4 alike) : Product  Inputs=2  SaturateOnIntegerOverflow=on
  Sum : Sum  Inputs=++  SaturateOnIntegerOverflow=on
  Sum1 : Sum  Inputs=++  SaturateOnIntegerOverflow=on
  Trigonometric Function : Trigonometry  Orientation=up  Operator=sin  OutputSignalType=auto
  cos (alpha) : Trigonometry  Operator=cos  OutputSignalType=auto
  cos (phi) : Trigonometry  Operator=cos  OutputSignalType=auto
  sen (phi) : Trigonometry  Operator=sin  OutputSignalType=auto
  x : Outport  Port=1  InitialOutput=0
  y : Outport  Port=2  InitialOutput=0
  phi : Outport  Port=3  InitialOutput=0
  wires:
  Product5/1 -> Sum/2, Sum1/2
  Integrator3/1 -> y/1
  Sum1/1 -> Integrator3/1
  Product6/1 -> Sum1/1
  Integrator2/1 -> x/1
  Sum/1 -> Integrator2/1
  Product4/1 -> Sum/1
  cos (phi)/1 -> Product6/1
  walpha/1 -> Product5/2, Integrator/1
  cos (alpha)/1 -> Product5/1
  sen (phi)/1 -> Product4/2
  Gain2/1 -> Product4/1
  Integrator1/1 -> cos (phi)/1, sen (phi)/1, phi/1
  Integrator/1 -> cos (alpha)/1, Trigonometric Function/1
  Gain/1 -> Product6/2, Product3/1, Gain2/1
  Product3/1 -> Integrator1/1
  Gain1/1 -> Product3/2
  Trigonometric Function/1 -> Gain1/1
  wt/1 -> Gain/1

== system HEMERO/Robots móviles/Modelos cinemáticos directos/Modelo directo Config. Síncrona ==
  note: phi
  note: x '
  note: phi'
  note: y '
  v : Inport  Port=1  PortWidth=-1  SampleTime=-1  DataType=auto
      settings: SignalType=auto
  w : Inport  Port=2  PortWidth=-1  SampleTime=-1  DataType=auto
      settings: SignalType=auto
  Gain2 : Gain  Gain=-1  SaturateOnIntegerOverflow=on
  Integrator : Integrator  ExternalReset=none  InitialConditionSource=internal  InitialCondition=phi_ini  LimitOutput=off  UpperSaturationLimit=inf  LowerSaturationLimit=-inf  ShowSaturationPort=off  ShowStatePort=off  AbsoluteTolerance=auto
  Integrator1 : Integrator  ExternalReset=none  InitialConditionSource=internal  InitialCondition=x_ini  LimitOutput=off  UpperSaturationLimit=inf  LowerSaturationLimit=-inf  ShowSaturationPort=off  ShowStatePort=off  AbsoluteTolerance=auto
  Integrator2 : Integrator  ExternalReset=none  InitialConditionSource=internal  InitialCondition=y_ini  LimitOutput=off  UpperSaturationLimit=inf  LowerSaturationLimit=-inf  ShowSaturationPort=off  ShowStatePort=off  AbsoluteTolerance=auto
  Product1 : Product  Inputs=2  SaturateOnIntegerOverflow=on
  Product2 : Product  Inputs=2  SaturateOnIntegerOverflow=on
  cos (phi) : Trigonometry  Operator=cos  OutputSignalType=auto
  sen (phi) : Trigonometry  Operator=sin  OutputSignalType=auto
  x : Outport  Port=1  InitialOutput=0
  y : Outport  Port=2  InitialOutput=0
  phi : Outport  Port=3  InitialOutput=0
  wires:
  Integrator/1 -> sen (phi)/1, cos (phi)/1, phi/1
  w/1 -> Integrator/1
  sen (phi)/1 -> Gain2/1
  Gain2/1 -> Product1/1
  Integrator1/1 -> x/1
  Product1/1 -> Integrator1/1
  cos (phi)/1 -> Product2/1
  v/1 -> Product1/2, Product2/2
  Integrator2/1 -> y/1
  Product2/1 -> Integrator2/1

== system HEMERO/Robots móviles/Modelos cinemáticos directos/Modelo directo Guiado Diferencial ==
  note: phi'
  note: x '
  note: y '
  note: phi
  wi : Inport  Port=1  PortWidth=-1  SampleTime=-1  DataType=auto
      settings: SignalType=auto
  wd : Inport  Port=2  PortWidth=-1  SampleTime=-1  DataType=auto
      settings: SignalType=auto
  Gain : Gain  Gain=c/b  SaturateOnIntegerOverflow=on
  Gain1 : Gain  Gain=c/2  SaturateOnIntegerOverflow=on
  Gain2 : Gain  Gain=-1  SaturateOnIntegerOverflow=on
  Integrator : Integrator  ExternalReset=none  InitialConditionSource=internal  InitialCondition=phi_ini  LimitOutput=off  UpperSaturationLimit=inf  LowerSaturationLimit=-inf  ShowSaturationPort=off  ShowStatePort=off  AbsoluteTolerance=auto
  Integrator1 : Integrator  ExternalReset=none  InitialConditionSource=internal  InitialCondition=x_ini  LimitOutput=off  UpperSaturationLimit=inf  LowerSaturationLimit=-inf  ShowSaturationPort=off  ShowStatePort=off  AbsoluteTolerance=auto
  Integrator2 : Integrator  ExternalReset=none  InitialConditionSource=internal  InitialCondition=y_ini  LimitOutput=off  UpperSaturationLimit=inf  LowerSaturationLimit=-inf  ShowSaturationPort=off  ShowStatePort=off  AbsoluteTolerance=auto
  Product : Product  Inputs=2  SaturateOnIntegerOverflow=on
  Product1 : Product  Inputs=2  SaturateOnIntegerOverflow=on
  Sum : Sum  Inputs=++  SaturateOnIntegerOverflow=on
  Sum1 : Sum  Inputs=-+  SaturateOnIntegerOverflow=on
  cos(phi) : Trigonometry  Operator=cos  OutputSignalType=auto
  sen(phi) : Trigonometry  Operator=sin  OutputSignalType=auto
  x : Outport  Port=1  InitialOutput=0
  y : Outport  Port=2  InitialOutput=0
  phi : Outport  Port=3  InitialOutput=0
  wires:
  wi/1 -> Sum/1, Sum1/1
  Sum/1 -> Gain1/1
  Gain1/1 -> Gain2/1, Product1/2
  Product1/1 -> Integrator2/1
  cos(phi)/1 -> Product1/1
  Product/1 -> Integrator1/1
  sen(phi)/1 -> Product/2
  Integrator1/1 -> x/1
  Integrator2/1 -> y/1
  wd/1 -> Sum1/2, Sum/2
  Sum1/1 -> Gain/1
  Gain/1 -> Integrator/1
  Integrator/1 -> sen(phi)/1, cos(phi)/1, phi/1
  Gain2/1 -> Product/1

== system HEMERO/Robots móviles/Modelos cinemáticos directos/Modelo directo Triciclo Clásico ==
  note: vt
  note: alpha
  note: phi
  wt : Inport  Port=1  PortWidth=-1  SampleTime=-1  DataType=auto
      settings: SignalType=auto
  walpha : Inport  Port=2  PortWidth=-1  SampleTime=-1  DataType=auto
      settings: SignalType=auto
  Gain : Gain  Gain=c  SaturateOnIntegerOverflow=on
  Gain1 : Gain  Orientation=up  Gain=1/l  SaturateOnIntegerOverflow=on
  Gain2 : Gain  Gain=-1  SaturateOnIntegerOverflow=on
  Integrator : Integrator  ExternalReset=none  InitialConditionSource=internal  InitialCondition=alpha_ini  LimitOutput=off  UpperSaturationLimit=inf  LowerSaturationLimit=-inf  ShowSaturationPort=off  ShowStatePort=off  AbsoluteTolerance=auto
  Integrator1 : Integrator  ExternalReset=none  InitialConditionSource=internal  InitialCondition=phi_ini  LimitOutput=off  UpperSaturationLimit=inf  LowerSaturationLimit=-inf  ShowSaturationPort=off  ShowStatePort=off  AbsoluteTolerance=auto
  Integrator2 : Integrator  ExternalReset=none  InitialConditionSource=internal  InitialCondition=x_ini  LimitOutput=off  UpperSaturationLimit=inf  LowerSaturationLimit=-inf  ShowSaturationPort=off  ShowStatePort=off  AbsoluteTolerance=auto
  Integrator3 : Integrator  ExternalReset=none  InitialConditionSource=internal  InitialCondition=y_ini  LimitOutput=off  UpperSaturationLimit=inf  LowerSaturationLimit=-inf  ShowSaturationPort=off  ShowStatePort=off  AbsoluteTolerance=auto
  Product{3..6} (4 alike) : Product  Inputs=2  SaturateOnIntegerOverflow=on
  Sum : Sum  Inputs=++  SaturateOnIntegerOverflow=on
  Sum1 : Sum  Inputs=++  SaturateOnIntegerOverflow=on
  Trigonometric Function : Trigonometry  Orientation=up  Operator=sin  OutputSignalType=auto
  cos (alpha) : Trigonometry  Operator=cos  OutputSignalType=auto
  cos (phi) : Trigonometry  Operator=cos  OutputSignalType=auto
  sen (phi) : Trigonometry  Operator=sin  OutputSignalType=auto
  x : Outport  Port=1  InitialOutput=0
  y : Outport  Port=2  InitialOutput=0
  phi : Outport  Port=3  InitialOutput=0
  wires:
  wt/1 -> Gain/1
  Trigonometric Function/1 -> Gain1/1
  Gain1/1 -> Product3/2
  Product3/1 -> Integrator1/1
  Gain/1 -> Gain2/1, Product3/1, Product6/2
  Integrator/1 -> Trigonometric Function/1, cos (alpha)/1
  Integrator1/1 -> phi/1, sen (phi)/1, cos (phi)/1
  Gain2/1 -> Product4/1
  sen (phi)/1 -> Product4/2
  cos (alpha)/1 -> Product5/1
  walpha/1 -> Integrator/1, Product5/2
  cos (phi)/1 -> Product6/1
  Product4/1 -> Sum/1
  Sum/1 -> Integrator2/1
  Integrator2/1 -> x/1
  Product6/1 -> Sum1/1
  Sum1/1 -> Integrator3/1
  Integrator3/1 -> y/1
  Product5/1 -> Sum1/2, Sum/2
